simulink model "EMT_G1"  (R2024a)
settings: Solver=ode1  StartTime=0.0  StopTime=simtime  FixedStep=Ts  RelTol=1e-3
values from neighbouring files (symbols this model uses):
  c0 = c0_hawk    (= 6.37282e-09)    [EMT_Phasor_parameters.m]
  c1 = c1_hawk    (= 8.76156e-09)    [EMT_Phasor_parameters.m]
  fg = 50    [EMT_Phasor_parameters.m]
  G1gen = 0.1245    [EMT_Phasor_parameters.m]
  G2gen = 0.30    (= 0.3)    [EMT_Phasor_parameters.m]
  G3gen = 0.20    (= 0.2)    [EMT_Phasor_parameters.m]
  G4sgen = 0.2078    [EMT_Phasor_parameters.m]
  G5gen = 0.20    (= 0.2)    [EMT_Phasor_parameters.m]
  G6gen = 0.2078    [EMT_Phasor_parameters.m]
  G6sgen = 0.20    (= 0.2)    [EMT_Phasor_parameters.m]
  G7gen = 0.518    [EMT_Phasor_parameters.m]
  Ihvpk = Ihv*sqrt(2)    [EMT_Phasor_parameters.m]
  l0 = l0_hawk    (= 0.00373)    [EMT_Phasor_parameters.m]
  l1 = l1_hawk    (= 0.00133)    [EMT_Phasor_parameters.m]
  L3dem = 0.10    (= 0.1)    [EMT_Phasor_parameters.m]
  L4dem = 0.30    (= 0.3)    [EMT_Phasor_parameters.m]
  L5dem = 0.35    [EMT_Phasor_parameters.m]
  L6dem = 0.15    [EMT_Phasor_parameters.m]
  L7dem = 0.10    (= 0.1)    [EMT_Phasor_parameters.m]
  Pr = Sr*PF    (= 550050000)    [EMT_Phasor_parameters.m]
  Qr = sqrt(Sr^2 - Pr^2)    [EMT_Phasor_parameters.m]
  r0 = r0_hawk    (= 0.44587)    [EMT_Phasor_parameters.m]
  r1 = r1_hawk    (= 0.12087)    [EMT_Phasor_parameters.m]
  Rtpu = Xtpu/40    (= 0.00375)    [EMT_Phasor_parameters.m]
  S1non = 400e6    (= 400000000)    [EMT_Phasor_parameters.m]
  S2non = 300e6    (= 300000000)    [EMT_Phasor_parameters.m]
  S3non = 200e6    (= 200000000)    [EMT_Phasor_parameters.m]
  S4snon = 200e6    (= 200000000)    [EMT_Phasor_parameters.m]
  S5non = 500e6    (= 500000000)    [EMT_Phasor_parameters.m]
  S6non = 400e6    (= 400000000)    [EMT_Phasor_parameters.m]
  S6snon = 200e6    (= 200000000)    [EMT_Phasor_parameters.m]
  S7non = 200e6    (= 200000000)    [EMT_Phasor_parameters.m]
  simtime = 5    [EMT_Phasor_parameters.m]
  tonvsc = 0.01    [EMT_Phasor_parameters.m]
  Ts = 150e-6    (= 0.00015)    [EMT_Phasor_parameters.m]
  Vhv = 220e3    (= 220000)    [EMT_Phasor_parameters.m]
  Vmv = 22e3    (= 22000)    [EMT_Phasor_parameters.m]
  wc1 = wsw1/10    (= 848.230016469)    [EMT_Phasor_parameters.m]
  wdc1 = wc1/10    (= 84.8230016469)    [EMT_Phasor_parameters.m]
  wpq1 = wc1/10    (= 84.8230016469)    [EMT_Phasor_parameters.m]
  wsw1 = ksw1*2*pi*fg    (= 8482.30016469)    [EMT_Phasor_parameters.m]
  Xtpu = 0.15    [EMT_Phasor_parameters.m]
undefined symbols (not defined in the file or in its folder): D11, Delta, Kf, r, theta0
libraries: simulink_extras x152, spsGroundLib x45, powerlib x40, spsCurrentMeasurementLib x39, spsVoltageMeasurementLib x33, simulink x32, eeGeneralControl x32, slpidlib x32, powerlib_meascontrol x28, spsFirstOrderFilterLib x24, eeTransforms x24, pid_lib x16
(part 4 of 16)

== system EMT_G1/G5/VSC ==
  note: If using different transformer connection,
      | compensate the delay in the modulation
  Block : Step  Time=0.02  Before=1  After=0  SampleTime=0
  NOT : Logic  Operator=NOT  IconShape=distinctive  AllPortsSameDT=off  OutDataTypeStr=boolean
  Pset : Step  Time=tonvsc  After=-S5non*G5gen  SampleTime=0
  Qset : Step  Time=tonvsc  After=-30e6  SampleTime=0
  Three-Phase Transformer (Two Windings) : spsThreePhaseTransformerTwoWindingsLib/Three-Phase Transformer (Two Windings)  Winding1Connection=Yg  Winding2Connection=Delta (D11)  CoreType=Three single-phase transformers  SetSaturation=off  Hysteresis=off  DataFile='hysteresis'  SetInitialFlux=off  Measurements=None  UNITS=pu  NominalPower=[Pconv , fg ]  Winding1=[Vhv, Rtpu/2, Xtpu/2]  Winding2=[Vmv, Rtpu/2, Xtpu/2]  Rm=5000  Lm=5000  L0=0.5  Saturation=[ 0,0 ; 0.0024,1.2 ; 1.0,1.52 ]  InitialFluxes=[ 0.8 , -0.8 , 0.7 ]  BreakLoop=off  DiscreteSolver=Trapezoidal iterative  DataType=off  TransfoNumber=1
  Three-Phase Breaker : spsThreePhaseBreakerLib/Three-Phase Breaker  InitialState=open  SwitchA=on  SwitchB=on  SwitchC=on  SwitchTimes="[1/60  5/60]"  External=on  BreakerResistance=0.001  SnubberResistance=1e7  SnubberCapacitance=inf  Measurements=None
  VI measurement : Subsystem
      settings: PortSchema="{\"entries\":[{\"content\":{\"sides\":[{\"content\":{\"connectorIds\":[\"LConn1\",\"LConn2\",\"LConn3\"]},\"type\":\"ConnectorPlacement.EquallySpacedRectSide\",\"uuid\":\"d0d5b0b8-afec-4f90-9eba-536a06b10059\"},{\"content\":{\"connectorIds\":[\"RConn1\",\"RConn2\",\"RConn3\"],\"side\":\"RIGHT\"},\"type\":\"ConnectorPlacement.EquallySpacedRectSide\",\"uuid\":\"adc1b68d-6172-4507-b54b-9373921355a1\"},{\"content\":{\"connectorIds\":[\"Out1\",\"Out2\"],\"side\":\"TOP\"},\"type\":\"ConnectorPlacement.EquallySpacedRectSide\",\"uuid\":\"8c5adf07-e95b-4907-94c3-1b2a47d47f40\"}]},\"type\":\"ConnectorPlacement.EquallySpacedConnector\",\"uuid\":\"87d0b20f-8f85-4790-a611-3415e642a83a\"}],\"packageUris\":[\"http://schema.mathworks.com/mf0/Connector/R2020b\"],\"version\":\"1.0\"}"
  VSC Control : Subsystem
      settings: PortSchema="{\"entries\":[{\"content\":{\"sides\":[{\"content\":{\"connectorIds\":[\"In1\",\"In2\",\"In3\",\"In4\",\"In5\"]},\"type\":\"ConnectorPlacement.EquallySpacedRectSide\",\"uuid\":\"cada8d9e-53e0-4197-9386-6c7b6ea13844\"},{\"content\":{\"connectorIds\":[\"Out1\"],\"side\":\"RIGHT\"},\"type\":\"ConnectorPlacement.EquallySpacedRectSide\",\"uuid\":\"f237b52a-0d77-45c0-937d-32cafba1283e\"},{\"content\":{\"connectorIds\":[\"Out2\"],\"side\":\"TOP\"},\"type\":\"ConnectorPlacement.EquallySpacedRectSide\",\"uuid\":\"e6f268b5-5f09-49a6-9529-b1aeebd5f021\"}]},\"type\":\"ConnectorPlacement.EquallySpacedConnector\",\"uuid\":\"4d1d2957-2eb9-4111-8c87-957e800b2b0b\"}],\"packageUris\":[\"http://schema.mathworks.com/mf0/Connector/19700101\"],\"version\":\"1.0\"}"
  VSC Model : Subsystem  Variant=on  VariantControlMode=label  LabelModeActiveChoice=EMT_AVG
      settings: PortSchema="{\"entries\":[{\"content\":{\"sides\":[{\"content\":{\"connectorIds\":[\"LConn1\",\"LConn2\",\"LConn3\"]},\"type\":\"ConnectorPlacement.EquallySpacedRectSide\",\"uuid\":\"96043b84-a665-4cb2-a938-d6633d7ee474\"},{\"content\":{\"connectorIds\":[\"In1\"],\"side\":\"RIGHT\"},\"type\":\"ConnectorPlacement.EquallySpacedRectSide\",\"uuid\":\"064d463f-c23a-42ac-89ce-8dea3d446214\"},{\"content\":{\"connectorIds\":[],\"side\":\"TOP\"},\"type\":\"ConnectorPlacement.EquallySpacedRectSide\",\"uuid\":\"95ef669c-c6ed-44c3-8b69-447906728b6d\"}]},\"type\":\"ConnectorPlacement.EquallySpacedConnector\",\"uuid\":\"ea66db09-64d7-4d7e-ba7b-d769c56e2dbd\"}],\"packageUris\":[\"http://schema.mathworks.com/mf0/Connector/19700101\"],\"version\":\"1.0\"}"
  output signals : Subsystem
  A : PMIOPort  Side=Left
  B : PMIOPort  Port=2  Side=Left
  C : PMIOPort  Port=3  Side=Left
  m : Outport
  wires:
  NOT/1 -> Three-Phase Breaker/1
  VSC Control/1(Ref) -> VSC Model/1(Ref)
  [Is] -> VSC Control/3(Iabc)
  [Vs] -> VSC Control/2(Vabc)
  Block/1 -> VSC Control/1(Block), NOT/1
  [Vs] -> output signals/1(Vs)
  [Is] -> output signals/2(Is)
  VSC Control/2(m) -> output signals/3(control)
  output signals/1(m) -> m/1
  VI measurement/1(Vs) -> [Vs]
  VI measurement/2(Is) -> [Is]
  Pset/1 -> VSC Control/4(Pset)
  Qset/1 -> VSC Control/5(Qset)
  connections:
  Three-Phase Transformer (Two Windings)/LConn3 -- Three-Phase Breaker/LConn3
  Three-Phase Transformer (Two Windings)/LConn2 -- Three-Phase Breaker/LConn2
  Three-Phase Transformer (Two Windings)/LConn1 -- Three-Phase Breaker/LConn1
  Three-Phase Transformer (Two Windings)/RConn3 -- VSC Model/LConn3
  Three-Phase Transformer (Two Windings)/RConn2 -- VSC Model/LConn2
  Three-Phase Transformer (Two Windings)/RConn1 -- VSC Model/LConn1
  Three-Phase Breaker/RConn1 -- VI measurement/RConn1
  Three-Phase Breaker/RConn2 -- VI measurement/RConn2
  Three-Phase Breaker/RConn3 -- VI measurement/RConn3
  VI measurement/LConn3 -- C/RConn1
  A/RConn1 -- VI measurement/LConn1
  B/RConn1 -- VI measurement/LConn2

== system EMT_G1/G6/VSC ==
  note: If using different transformer connection,
      | compensate the delay in the modulation
  Block : Step  Time=0.02  Before=1  After=0  SampleTime=0
  NOT : Logic  Operator=NOT  IconShape=distinctive  AllPortsSameDT=off  OutDataTypeStr=boolean
  Pset : Step  Time=tonvsc  After=-S6non*G6gen  SampleTime=0
  Qset : Step  Time=tonvsc  After=-30e6  SampleTime=0
  Three-Phase Transformer (Two Windings) : spsThreePhaseTransformerTwoWindingsLib/Three-Phase Transformer (Two Windings)  Winding1Connection=Yg  Winding2Connection=Delta (D11)  CoreType=Three single-phase transformers  SetSaturation=off  Hysteresis=off  DataFile='hysteresis'  SetInitialFlux=off  Measurements=None  UNITS=pu  NominalPower=[Pconv , fg ]  Winding1=[Vhv, Rtpu/2, Xtpu/2]  Winding2=[Vmv, Rtpu/2, Xtpu/2]  Rm=5000  Lm=5000  L0=0.5  Saturation=[ 0,0 ; 0.0024,1.2 ; 1.0,1.52 ]  InitialFluxes=[ 0.8 , -0.8 , 0.7 ]  BreakLoop=off  DiscreteSolver=Trapezoidal iterative  DataType=off  TransfoNumber=1
  Three-Phase Breaker : spsThreePhaseBreakerLib/Three-Phase Breaker  InitialState=open  SwitchA=on  SwitchB=on  SwitchC=on  SwitchTimes="[1/60  5/60]"  External=on  BreakerResistance=0.001  SnubberResistance=1e7  SnubberCapacitance=inf  Measurements=None
  VI measurement : Subsystem
      settings: PortSchema="{\"entries\":[{\"content\":{\"sides\":[{\"content\":{\"connectorIds\":[\"LConn1\",\"LConn2\",\"LConn3\"]},\"type\":\"ConnectorPlacement.EquallySpacedRectSide\",\"uuid\":\"d0d5b0b8-afec-4f90-9eba-536a06b10059\"},{\"content\":{\"connectorIds\":[\"RConn1\",\"RConn2\",\"RConn3\"],\"side\":\"RIGHT\"},\"type\":\"ConnectorPlacement.EquallySpacedRectSide\",\"uuid\":\"adc1b68d-6172-4507-b54b-9373921355a1\"},{\"content\":{\"connectorIds\":[\"Out1\",\"Out2\"],\"side\":\"TOP\"},\"type\":\"ConnectorPlacement.EquallySpacedRectSide\",\"uuid\":\"8c5adf07-e95b-4907-94c3-1b2a47d47f40\"}]},\"type\":\"ConnectorPlacement.EquallySpacedConnector\",\"uuid\":\"87d0b20f-8f85-4790-a611-3415e642a83a\"}],\"packageUris\":[\"http://schema.mathworks.com/mf0/Connector/R2020b\"],\"version\":\"1.0\"}"
  VSC Control : Subsystem
      settings: PortSchema="{\"entries\":[{\"content\":{\"sides\":[{\"content\":{\"connectorIds\":[\"In1\",\"In2\",\"In3\",\"In4\",\"In5\"]},\"type\":\"ConnectorPlacement.EquallySpacedRectSide\",\"uuid\":\"cada8d9e-53e0-4197-9386-6c7b6ea13844\"},{\"content\":{\"connectorIds\":[\"Out1\"],\"side\":\"RIGHT\"},\"type\":\"ConnectorPlacement.EquallySpacedRectSide\",\"uuid\":\"f237b52a-0d77-45c0-937d-32cafba1283e\"},{\"content\":{\"connectorIds\":[\"Out2\"],\"side\":\"TOP\"},\"type\":\"ConnectorPlacement.EquallySpacedRectSide\",\"uuid\":\"e6f268b5-5f09-49a6-9529-b1aeebd5f021\"}]},\"type\":\"ConnectorPlacement.EquallySpacedConnector\",\"uuid\":\"4d1d2957-2eb9-4111-8c87-957e800b2b0b\"}],\"packageUris\":[\"http://schema.mathworks.com/mf0/Connector/19700101\"],\"version\":\"1.0\"}"
  VSC Model : Subsystem  Variant=on  VariantControlMode=label  LabelModeActiveChoice=EMT_AVG
      settings: PortSchema="{\"entries\":[{\"content\":{\"sides\":[{\"content\":{\"connectorIds\":[\"LConn1\",\"LConn2\",\"LConn3\"]},\"type\":\"ConnectorPlacement.EquallySpacedRectSide\",\"uuid\":\"96043b84-a665-4cb2-a938-d6633d7ee474\"},{\"content\":{\"connectorIds\":[\"In1\"],\"side\":\"RIGHT\"},\"type\":\"ConnectorPlacement.EquallySpacedRectSide\",\"uuid\":\"064d463f-c23a-42ac-89ce-8dea3d446214\"},{\"content\":{\"connectorIds\":[],\"side\":\"TOP\"},\"type\":\"ConnectorPlacement.EquallySpacedRectSide\",\"uuid\":\"95ef669c-c6ed-44c3-8b69-447906728b6d\"}]},\"type\":\"ConnectorPlacement.EquallySpacedConnector\",\"uuid\":\"ea66db09-64d7-4d7e-ba7b-d769c56e2dbd\"}],\"packageUris\":[\"http://schema.mathworks.com/mf0/Connector/19700101\"],\"version\":\"1.0\"}"
  output signals : Subsystem
  A : PMIOPort  Side=Left
  B : PMIOPort  Port=2  Side=Left
  C : PMIOPort  Port=3  Side=Left
  m : Outport
  wires:
  NOT/1 -> Three-Phase Breaker/1
  VSC Control/1(Ref) -> VSC Model/1(Ref)
  [Is] -> VSC Control/3(Iabc)
  [Vs] -> VSC Control/2(Vabc)
  Block/1 -> VSC Control/1(Block), NOT/1
  [Vs] -> output signals/1(Vs)
  [Is] -> output signals/2(Is)
  VSC Control/2(m) -> output signals/3(control)
  output signals/1(m) -> m/1
  VI measurement/1(Vs) -> [Vs]
  VI measurement/2(Is) -> [Is]
  Pset/1 -> VSC Control/4(Pset)
  Qset/1 -> VSC Control/5(Qset)
  connections:
  Three-Phase Transformer (Two Windings)/LConn3 -- Three-Phase Breaker/LConn3
  Three-Phase Transformer (Two Windings)/LConn2 -- Three-Phase Breaker/LConn2
  Three-Phase Transformer (Two Windings)/LConn1 -- Three-Phase Breaker/LConn1
  Three-Phase Transformer (Two Windings)/RConn3 -- VSC Model/LConn3
  Three-Phase Transformer (Two Windings)/RConn2 -- VSC Model/LConn2
  Three-Phase Transformer (Two Windings)/RConn1 -- VSC Model/LConn1
  Three-Phase Breaker/RConn1 -- VI measurement/RConn1
  Three-Phase Breaker/RConn2 -- VI measurement/RConn2
  Three-Phase Breaker/RConn3 -- VI measurement/RConn3
  VI measurement/LConn3 -- C/RConn1
  A/RConn1 -- VI measurement/LConn1
  B/RConn1 -- VI measurement/LConn2

== system EMT_G1/G6s/Exciter System ==
  <dw> : Inport
  Vref : Inport  Port=2
  Vt : Inport  Port=3
  It : Inport  Port=4
  <Peo> : Inport  Port=5
  PSS : Subsystem  mask{Ks1=10, Ks2=0.1564, Ks3=1, Tw1=2, Tw2=2, Tw3=2, Tw4=0, T1=0.25, T2=0.03, T3=0.15, T4=0.015, T6=0, T7=2, T8=0.5, T9=0.1, Vstmin=-0.1, Vstmax=0.1, N=0, M=0, IC1=1, IC2=3}
      mask prompts: Ks1 "PSS gain (Ks1)"; Ks2 "2nd signal transducer factor(Ks2)"; Ks3 "washouts coupling factor (Ks3)"; Tw1 "1st washout 1th time constant (Tw1)(sec)"; Tw2 "1st washout 2nd time constant (Tw2)(sec)"; Tw3 "2nd washout 1st time constant (Tw3)(sec)"; Tw4 "2nd washout 2nd time constant (Tw4)(sec)"; T1 "1st lead-lag derivative time constant (T1)(sec)"; T2 "1st lead-lag delay time constant(T2)(sec)"; T3 "2nd lead-lag derivative time constant(T3)(sec)"; T4 "2nd lead-lag delay time constant(T4)(sec)"; T6 "1st signal transducer time constant(T6)(sec)"; T7 "2nd signal transducer time constant(T7)(sec)"; T8 "ramp tracking filter deriv. time constant(T8)(sec)"; T9 "ramp tracking filter delay time constant(T9)(sec)"; Vstmin "controller minimum output(Vstmin)"; Vstmax "controller maximum output(Vstmax)"; N "ramp tracking filter (N)"; M "ramp tracking filter (M)"; IC1 "1st input selector (IC1)"; IC2 "2nd input selector (IC2)"
      mask Display:
      | disp('PSS2A')
      | 
      | port_label('input',1,'dw')
      | port_label('input',2,'Pg')
      | %port_label('input',3,'Vs')
      | 
      | port_label('output',1,'Vs')
  SEXS : Subsystem  mask{K=200, Ta=3, Tb=10, Te=0.05, Emin=-4, Emax=4, Vf0=1.68751}
      mask prompts: K "Controller gain (K)"; Ta "Filter derivative time constant (Ta)(sec)"; Tb "Filter delay time (Tb)(sec)"; Te "Exciter time constant (Te)(sec)"; Emin "Controller minimum output (Emin)"; Emax "Controller maximum output (Emax)"; Vf0 "Initial output (p.u)"
      mask Display:
      | disp('AVR')
      | 
      | port_label('input',1,'Vref')
      | port_label('input',2,'Vc')
      | port_label('input',3,'Vs')
      | 
      | port_label('output',1,'Efd')
  TR and LC_test : Subsystem  mask{Tr=1e-3, Rc=0, Xc=0}
      mask prompts: Tr "Transducter filter time constant (Tr)(sec)"; Rc "Resistance to compensate (p.u)"; Xc "Reactance to compensate (p.u)"
      mask Display:
      | %disp('Transducer \n \n')
      | %disp('and \n')
      | %disp('Load compensation')
      | text(15,35, 'Transducer')
      | text(30,24, 'and')
      | text(15,14, 'Load comp')
      | 
      | port_label('input',1,'Vt')
      | port_label('input',2,'It')
      | 
      | port_label('output',1,'Vc')
  Efd : Outport
  wires:
  SEXS/1(Efd) -> Efd/1
  It/1 -> TR and LC_test/2(It)
  PSS/1(Vothsg) -> SEXS/3(Vs)
  <Peo>/1 -> PSS/2(Pgen)
  <dw>/1 -> PSS/1(dw)
  Vt/1 -> TR and LC_test/1(Vt)
  Vref/1 -> SEXS/1(Vref)
  TR and LC_test/1(Vc) -> SEXS/2(Vc)

== system EMT_G1/G6s/Speed Governor ==
  note: mechanical power
  RefL : Inport
  dw : Inport  Port=2
  Gain1 : Gain  Gain=Dt
  Gain2 : Gain  Gain=1/R
  Saturation : Saturate  UpperLimit=Vmax  LowerLimit=Vmin
  Saturation1 : Saturate  UpperLimit=1
  Scope : Scope  NumInputPorts=2
  Sum : Sum  Inputs=|+-
  Sum1 : Sum  Inputs=|+-
  Transfer Fcn (with initial outputs)1 : simulink_extras/Additional Linear/Transfer Fcn (with initial outputs)  N=[T2 1]  D=[T3 1]  Y0=P0  U0=P0
  Transfer Fcn (with initial outputs)2 : simulink_extras/Additional Linear/Transfer Fcn (with initial outputs)  N=[1]  D=[T1 1]  Y0=P0  U0=P0
  Pm : Outport
  wires:
  Gain2/1 -> Sum/2
  dw/1 -> Gain2/1, Gain1/1
  Gain1/1 -> Sum1/2
  Transfer Fcn (with initial outputs)1/1 -> Sum1/1
  Sum1/1 -> Saturation1/1
  Saturation/1 -> Scope/1, Transfer Fcn (with initial outputs)1/1
  Transfer Fcn (with initial outputs)2/1 -> Saturation/1
  Sum/1 -> Transfer Fcn (with initial outputs)2/1
  RefL/1 -> Sum/1
  Saturation1/1 -> Scope/2, Pm/1

== system EMT_G1/G7/Exciter System ==
  <dw> : Inport
  Vref : Inport  Port=2
  Vt : Inport  Port=3
  It : Inport  Port=4
  <Peo> : Inport  Port=5
  PSS1 : Subsystem  mask{Ks1=10, Ks2=0.1564, Ks3=1, Tw1=2, Tw2=2, Tw3=2, Tw4=0, T1=0.25, T2=0.03, T3=0.15, T4=0.015, T6=0, T7=2, T8=0.5, T9=0.1, Vstmin=-0.1, Vstmax=0.1, N=0, M=0, IC1=1, IC2=3}
      mask prompts: Ks1 "PSS gain (Ks1)"; Ks2 "2nd signal transducer factor(Ks2)"; Ks3 "washouts coupling factor (Ks3)"; Tw1 "1st washout 1th time constant (Tw1)(sec)"; Tw2 "1st washout 2nd time constant (Tw2)(sec)"; Tw3 "2nd washout 1st time constant (Tw3)(sec)"; Tw4 "2nd washout 2nd time constant (Tw4)(sec)"; T1 "1st lead-lag derivative time constant (T1)(sec)"; T2 "1st lead-lag delay time constant(T2)(sec)"; T3 "2nd lead-lag derivative time constant(T3)(sec)"; T4 "2nd lead-lag delay time constant(T4)(sec)"; T6 "1st signal transducer time constant(T6)(sec)"; T7 "2nd signal transducer time constant(T7)(sec)"; T8 "ramp tracking filter deriv. time constant(T8)(sec)"; T9 "ramp tracking filter delay time constant(T9)(sec)"; Vstmin "controller minimum output(Vstmin)"; Vstmax "controller maximum output(Vstmax)"; N "ramp tracking filter (N)"; M "ramp tracking filter (M)"; IC1 "1st input selector (IC1)"; IC2 "2nd input selector (IC2)"
      mask Display:
      | disp('PSS2A')
      | 
      | port_label('input',1,'dw')
      | port_label('input',2,'Pg')
      | %port_label('input',3,'Vs')
      | 
      | port_label('output',1,'Vs')
  SEXS : Subsystem  mask{K=200, Ta=3, Tb=10, Te=0.05, Emin=-4, Emax=4, Vf0=1.77627}
      mask prompts: K "Controller gain (K)"; Ta "Filter derivative time constant (Ta)(sec)"; Tb "Filter delay time (Tb)(sec)"; Te "Exciter time constant (Te)(sec)"; Emin "Controller minimum output (Emin)"; Emax "Controller maximum output (Emax)"; Vf0 "Initial output (p.u)"
      mask Display:
      | disp('AVR')
      | 
      | port_label('input',1,'Vref')
      | port_label('input',2,'Vc')
      | port_label('input',3,'Vs')
      | 
      | port_label('output',1,'Efd')
  TR and LC_test : Subsystem  mask{Tr=1e-3, Rc=0, Xc=0}
      mask prompts: Tr "Transducter filter time constant (Tr)(sec)"; Rc "Resistance to compensate (p.u)"; Xc "Reactance to compensate (p.u)"
      mask Display:
      | %disp('Transducer \n \n')
      | %disp('and \n')
      | %disp('Load compensation')
      | text(15,35, 'Transducer')
      | text(30,24, 'and')
      | text(15,14, 'Load comp')
      | 
      | port_label('input',1,'Vt')
      | port_label('input',2,'It')
      | 
      | port_label('output',1,'Vc')
  Efd : Outport
  wires:
  TR and LC_test/1(Vc) -> SEXS/2(Vc)
  Vref/1 -> SEXS/1(Vref)
  Vt/1 -> TR and LC_test/1(Vt)
  <dw>/1 -> PSS1/1(dw)
  <Peo>/1 -> PSS1/2(Pgen)
  PSS1/1(Vothsg) -> SEXS/3(Vs)
  It/1 -> TR and LC_test/2(It)
  SEXS/1(Efd) -> Efd/1

== system EMT_G1/G7/Speed Governor ==
  note: mechanical power
  RefL : Inport
  dw : Inport  Port=2
  Gain1 : Gain  Gain=Dt
  Gain2 : Gain  Gain=1/R
  Saturation : Saturate  UpperLimit=Vmax  LowerLimit=Vmin
  Saturation1 : Saturate  UpperLimit=1
  Sum : Sum  Inputs=|+-
  Sum1 : Sum  Inputs=|+-
  Transfer Fcn (with initial outputs)1 : simulink_extras/Additional Linear/Transfer Fcn (with initial outputs)  N=[T2 1]  D=[T3 1]  Y0=P0  U0=P0
  Transfer Fcn (with initial outputs)2 : simulink_extras/Additional Linear/Transfer Fcn (with initial outputs)  N=[1]  D=[T1 1]  Y0=P0  U0=P0
  Pm : Outport
  wires:
  Saturation1/1 -> Pm/1
  RefL/1 -> Sum/1
  Sum/1 -> Transfer Fcn (with initial outputs)2/1
  Transfer Fcn (with initial outputs)2/1 -> Saturation/1
  Saturation/1 -> Transfer Fcn (with initial outputs)1/1
  Sum1/1 -> Saturation1/1
  Transfer Fcn (with initial outputs)1/1 -> Sum1/1
  Gain1/1 -> Sum1/2
  dw/1 -> Gain1/1, Gain2/1
  Gain2/1 -> Sum/2

== system EMT_G1/G1/Exciter System/PSS1 ==
  note: Power System Stabilizer (PSS2A)
  dw : Inport
  Pgen : Inport  Port=2
  Gain : Gain  Gain=Ks1
  Gain1 : Gain  Gain=Ks3
  Saturation : Saturate  UpperLimit=Vstmax  LowerLimit=Vstmin
  Sum1 : Sum  Inputs=|++
  Sum2 : Sum  Inputs=|+-
  Transfer Fcn1 : TransferFcn  Numerator=[Tw1 0]  Denominator=[Tw1 1]
  Transfer Fcn2 : TransferFcn  Numerator=[Tw3 0]  Denominator=[Tw3 1]
  Transfer Fcn3 : TransferFcn  Numerator=[Tw2 0]  Denominator=[Tw2 1]
  Transfer Fcn4 : TransferFcn  Denominator=[T6 1]
  Transfer Fcn5 : TransferFcn  Numerator=[T8 1].^N  Denominator=[T9 1].^(M*N)
  Transfer Fcn6 : TransferFcn  Numerator=[T1 1]  Denominator=[T2 1]
  Transfer Fcn7 : TransferFcn  Numerator=[T3 1]  Denominator=[T4 1]
  Transfer Fcn8 : TransferFcn  Numerator=[Tw4 0]  Denominator=[Tw4 1]
  Transfer Fcn9 : TransferFcn  Numerator=[Ks2]  Denominator=[T7 1]
  Vothsg : Outport
  wires:
  dw/1 -> Transfer Fcn1/1
  Transfer Fcn1/1 -> Transfer Fcn3/1
  Transfer Fcn3/1 -> Transfer Fcn4/1
  Transfer Fcn4/1 -> Sum1/1
  Sum1/1 -> Transfer Fcn5/1
  Transfer Fcn5/1 -> Sum2/1
  Sum2/1 -> Gain/1
  Gain/1 -> Transfer Fcn6/1
  Transfer Fcn6/1 -> Transfer Fcn7/1
  Transfer Fcn7/1 -> Saturation/1
  Saturation/1 -> Vothsg/1
  Pgen/1 -> Transfer Fcn2/1
  Transfer Fcn2/1 -> Transfer Fcn8/1
  Transfer Fcn8/1 -> Transfer Fcn9/1
  Gain1/1 -> Sum1/2
  Transfer Fcn9/1 -> Gain1/1, Sum2/2

== system EMT_G1/G1/Exciter System/PSS1 backup ==
  note: Power System Stabilizer (PSS2A)
  dw : Inport
  Pgen : Inport  Port=2
  Gain : Gain  Gain=Ks1
  Gain1 : Gain  Gain=Ks3
  Saturation : Saturate  UpperLimit=Vstmax  LowerLimit=Vstmin
  Sum1 : Sum  Inputs=|++
  Sum2 : Sum  Inputs=|+-
  Transfer Fcn1 : TransferFcn  Numerator=[Tw1 0]  Denominator=[Tw1 1]
  Transfer Fcn2 : TransferFcn  Numerator=[Tw3 0]  Denominator=[Tw3 1]
  Transfer Fcn3 : TransferFcn  Numerator=[Tw2 0]  Denominator=[Tw2 1]
  Transfer Fcn4 : TransferFcn  Denominator=[T6 1]
  Transfer Fcn5 : TransferFcn  Numerator=[T8 1].^N  Denominator=[T9 1].^(M*N)
  Transfer Fcn6 : TransferFcn  Numerator=[T1 1]  Denominator=[T2 1]
  Transfer Fcn7 : TransferFcn  Numerator=[T3 1]  Denominator=[T4 1]
  Transfer Fcn8 : TransferFcn  Numerator=[Tw4 0]  Denominator=[Tw4 1]
  Transfer Fcn9 : TransferFcn  Numerator=[Ks2]  Denominator=[T7 1]
  Vothsg : Outport
  wires:
  Transfer Fcn9/1 -> Sum2/2, Gain1/1
  Gain1/1 -> Sum1/2
  Transfer Fcn8/1 -> Transfer Fcn9/1
  Transfer Fcn2/1 -> Transfer Fcn8/1
  Pgen/1 -> Transfer Fcn2/1
  Saturation/1 -> Vothsg/1
  Transfer Fcn7/1 -> Saturation/1
  Transfer Fcn6/1 -> Transfer Fcn7/1
  Gain/1 -> Transfer Fcn6/1
  Sum2/1 -> Gain/1
  Transfer Fcn5/1 -> Sum2/1
  Sum1/1 -> Transfer Fcn5/1
  Transfer Fcn4/1 -> Sum1/1
  Transfer Fcn3/1 -> Transfer Fcn4/1
  Transfer Fcn1/1 -> Transfer Fcn3/1
  dw/1 -> Transfer Fcn1/1

== system EMT_G1/G1/Exciter System/SEXS ==
  note: The controller parameters provided by ENTSO-E
      | define different names for the parameters:
      |
      | ENTSO-E = IEEE Std 421.5-2005
      | Ta = Tc
      | Tb = Tb
      | K = Ka
      | Te = Ta
      | Emax = Vrmax
      | Emin = Vrmin
  note: The exciter model provided by ENTSO-E most similar to the IEEE is the Type AC4A excitation system model
  Vref : Inport
  Vc : Inport  Port=2
  Vs : Inport  Port=3
  1st ord transfer fcn windup limiter : Subsystem  mask{Gain=K, tau=Te, Vmax=Emax, Vmin=Emin, y0=Vf0}
      mask prompts: tau "Time constant"; y0 "Initial output"
  Constant : Constant  Value=Vf0/K
  Saturation : Saturate  Commented=through  UpperLimit=0.1  LowerLimit=-0.1
  Sum : Sum  Inputs=+-+
  Sum1 : Sum  Inputs=|++
  Transfer Fcn (with initial outputs)1 : simulink_extras/Additional Linear/Transfer Fcn (with initial outputs)  N=[Ta 1]  D=[Tb 1]  Y0=Vf0/K  U0=Vf0/K
  Efd : Outport
  wires:
  1st ord transfer fcn windup limiter/1(Out1) -> Efd/1
  Vs/1 -> Sum/3
  Vref/1 -> Sum/1
  Vc/1 -> Sum/2
  Transfer Fcn (with initial outputs)1/1 -> 1st ord transfer fcn windup limiter/1(In1)
  Saturation/1 -> Transfer Fcn (with initial outputs)1/1
  Sum/1 -> Sum1/1
  Sum1/1 -> Saturation/1
  Constant/1 -> Sum1/2

== system EMT_G1/G1/Exciter System/TR and LC_test ==
  note: Terminal voltage transducer and optional load compensation
  note: compensated
      | impedance
  note: Vt and It should be phasors (complex quantities)
  note: Fig 4.1 of IEEE Std 421.5-2005
  note: Rc and Xc should be negative values in case of voltage regulated after an impedance
  Vt : Inport
  It : Inport  Port=2
  Abs : Abs  SaturateOnIntegerOverflow=off
  Abs1 : Abs  SaturateOnIntegerOverflow=off
  Rc+jXc : Gain  Gain=abs(Rc+1i*Xc)
  Saturation : Saturate  UpperLimit=1.2  LowerLimit=0.8
  Sum : Sum  Inputs=|+-
  Transfer Fcn (with initial outputs) : simulink_extras/Additional Linear/Transfer Fcn (with initial outputs)  Commented=through  N=[1]  D=[Tr 1]  Y0=1  U0=1
  Vc : Outport
  wires:
  Saturation/1 -> Vc/1
  Vt/1 -> Abs/1
  Transfer Fcn (with initial outputs)/1 -> Saturation/1
  Rc+jXc/1 -> Sum/2
  Sum/1 -> Transfer Fcn (with initial outputs)/1
  It/1 -> Abs1/1
  Abs/1 -> Sum/1
  Abs1/1 -> Rc+jXc/1

== system EMT_G1/G2/VSC/VI measurement ==
  Current Measurement : spsCurrentMeasurementLib/Current Measurement  PhasorSimulation=off  OutputType=Complex  PSBequivalent=0
  Current Measurement1 : spsCurrentMeasurementLib/Current Measurement  PhasorSimulation=off  OutputType=Complex  PSBequivalent=0
  Current Measurement2 : spsCurrentMeasurementLib/Current Measurement  PhasorSimulation=off  OutputType=Complex  PSBequivalent=0
  Ground : spsGroundLib/Ground  LConnTagsString=a
  Ground1 : spsGroundLib/Ground  LConnTagsString=a
  Ground2 : spsGroundLib/Ground  LConnTagsString=a
  Mux : Mux  Inputs=3
  Mux1 : Mux  Inputs=3
  Voltage Measurement : spsVoltageMeasurementLib/Voltage Measurement  PhasorSimulation=off  OutputType=Complex  PSBequivalent=0
  Voltage Measurement1 : spsVoltageMeasurementLib/Voltage Measurement  PhasorSimulation=off  OutputType=Complex  PSBequivalent=0
  Voltage Measurement2 : spsVoltageMeasurementLib/Voltage Measurement  PhasorSimulation=off  OutputType=Complex  PSBequivalent=0
  A : PMIOPort  Side=Left
  B : PMIOPort  Port=2  Side=Left
  C : PMIOPort  Port=3  Side=Left
  a : PMIOPort  Port=4  Side=Right
  b : PMIOPort  Port=5  Side=Right
  c : PMIOPort  Port=6  Side=Right
  Vs : Outport
  Is : Outport  Port=2
  wires:
  Mux1/1 -> Is/1
  Mux/1 -> Vs/1
  Voltage Measurement1/1 -> Mux/2
  Voltage Measurement2/1 -> Mux/3
  Current Measurement2/1 -> Mux1/3
  Voltage Measurement/1 -> Mux/1
  Current Measurement/1 -> Mux1/1
  Current Measurement1/1 -> Mux1/2
  connections:
  Voltage Measurement/LConn1 -- Current Measurement/LConn1 -- A/RConn1
  Current Measurement2/LConn1 -- C/RConn1 -- Voltage Measurement2/LConn1
  Current Measurement1/LConn1 -- Voltage Measurement1/LConn1 -- B/RConn1
  Current Measurement1/RConn1 -- b/RConn1
  Current Measurement/RConn1 -- a/RConn1
  Ground/LConn1 -- Voltage Measurement/LConn2
  Current Measurement2/RConn1 -- c/RConn1
  Ground1/LConn1 -- Voltage Measurement1/LConn2
  Ground2/LConn1 -- Voltage Measurement2/LConn2

== system EMT_G1/G2/VSC/VSC Control ==
  Block : Inport
  Vabc : Inport  Port=2
  Iabc : Inport  Port=3
  Pset : Inport  Port=4
  Qset : Inport  Port=5
  Control loops : Subsystem  Variant=on  VariantControlMode=label  LabelModeActiveChoice=EMT_and_QEMT
  Measurements : Subsystem  Variant=on  VariantControlMode=label  LabelModeActiveChoice=EMT
  Modulation : Subsystem  Variant=on  VariantControlMode=label  LabelModeActiveChoice=EMT_AVG
  Mux : Mux  Inputs=2
  Ref : Outport
  m : Outport  Port=2
  wires:
  Control loops/2(iqd+-ref) -> Modulation/3(iqd+-*)
  Control loops/1(vqd+-ref) -> Modulation/2(vqd+-*)
  [PQabc] -> Mux/2
  Measurements/5(PQabc) -> [PQabc]
  Modulation/1(Ref) -> Ref/1
  Measurements/4(theta) -> [theta]
  Vabc/1 -> Measurements/1(Vabc)
  Measurements/1(vqd+-) -> Control loops/3(vqd+-), [vqdpn]
  Measurements/2(iqd+-) -> Control loops/4(iqd+-)
  Measurements/3(freq) -> Control loops/5(freq)
  [theta] -> Modulation/4(theta)
  [vqdpn] -> Modulation/1(vqd+-)
  Iabc/1 -> Measurements/2(Iabc)
  Mux/1 -> m/1
  Control loops/3(m) -> Mux/1
  Pset/1 -> Control loops/1(Pset)
  Qset/1 -> Control loops/2(Qset)
  Block/1 -> Control loops/6(Block)

== system EMT_G1/G2/VSC/VSC Model ==
  Ref : Inport
  EMT AVG : Subsystem  VariantControl=EMT_AVG
      settings: PortSchema="{\"entries\":[{\"content\":{\"sides\":[{\"content\":{\"connectorIds\":[\"LConn1\",\"LConn2\",\"LConn3\"]},\"type\":\"ConnectorPlacement.EquallySpacedRectSide\",\"uuid\":\"96043b84-a665-4cb2-a938-d6633d7ee474\"},{\"content\":{\"connectorIds\":[\"In1\"],\"side\":\"RIGHT\"},\"type\":\"ConnectorPlacement.EquallySpacedRectSide\",\"uuid\":\"064d463f-c23a-42ac-89ce-8dea3d446214\"},{\"content\":{\"connectorIds\":[],\"side\":\"TOP\"},\"type\":\"ConnectorPlacement.EquallySpacedRectSide\",\"uuid\":\"95ef669c-c6ed-44c3-8b69-447906728b6d\"}]},\"type\":\"ConnectorPlacement.EquallySpacedConnector\",\"uuid\":\"ea66db09-64d7-4d7e-ba7b-d769c56e2dbd\"}],\"packageUris\":[\"http://schema.mathworks.com/mf0/Connector/19700101\"],\"version\":\"1.0\"}"
  EMT SW : Subsystem  VariantControl=EMT_SW
      settings: PortSchema="{\"entries\":[{\"content\":{\"sides\":[{\"content\":{\"connectorIds\":[\"LConn1\",\"LConn2\",\"LConn3\"]},\"type\":\"ConnectorPlacement.EquallySpacedRectSide\",\"uuid\":\"96043b84-a665-4cb2-a938-d6633d7ee474\"},{\"content\":{\"connectorIds\":[\"In1\"],\"side\":\"RIGHT\"},\"type\":\"ConnectorPlacement.EquallySpacedRectSide\",\"uuid\":\"064d463f-c23a-42ac-89ce-8dea3d446214\"},{\"content\":{\"connectorIds\":[],\"side\":\"TOP\"},\"type\":\"ConnectorPlacement.EquallySpacedRectSide\",\"uuid\":\"95ef669c-c6ed-44c3-8b69-447906728b6d\"}]},\"type\":\"ConnectorPlacement.EquallySpacedConnector\",\"uuid\":\"ea66db09-64d7-4d7e-ba7b-d769c56e2dbd\"}],\"packageUris\":[\"http://schema.mathworks.com/mf0/Connector/19700101\"],\"version\":\"1.0\"}"
  Phasor : Subsystem  VariantControl=Phasor
      settings: PortSchema="{\"entries\":[{\"content\":{\"sides\":[{\"content\":{\"connectorIds\":[\"LConn1\",\"LConn2\",\"LConn3\"]},\"type\":\"ConnectorPlacement.EquallySpacedRectSide\",\"uuid\":\"96043b84-a665-4cb2-a938-d6633d7ee474\"},{\"content\":{\"connectorIds\":[\"In1\"],\"side\":\"RIGHT\"},\"type\":\"ConnectorPlacement.EquallySpacedRectSide\",\"uuid\":\"064d463f-c23a-42ac-89ce-8dea3d446214\"},{\"content\":{\"connectorIds\":[],\"side\":\"TOP\"},\"type\":\"ConnectorPlacement.EquallySpacedRectSide\",\"uuid\":\"95ef669c-c6ed-44c3-8b69-447906728b6d\"}]},\"type\":\"ConnectorPlacement.EquallySpacedConnector\",\"uuid\":\"ea66db09-64d7-4d7e-ba7b-d769c56e2dbd\"}],\"packageUris\":[\"http://schema.mathworks.com/mf0/Connector/19700101\"],\"version\":\"1.0\"}"
  A : PMIOPort  Side=Left
  B : PMIOPort  Port=2  Side=Left
  C : PMIOPort  Port=3  Side=Left

== system EMT_G1/G2/VSC/output signals ==
  Vs : Inport
  Is : Inport  Port=2
  control : Inport  Port=3
  Bus Creator : BusCreator  Inputs=15
  Demux : Demux  Outputs=13
  m : Outport
  wires:
  Bus Creator/1 -> m/1
  control/1 -> Demux/1
  Vs/1 -> Bus Creator/1  "Vabc"
  Is/1 -> Bus Creator/2  "Iabc"
  Demux/1 -> Bus Creator/3  "vqp"
  Demux/2 -> Bus Creator/4  "vdp"
  Demux/3 -> Bus Creator/5  "vqn"
  Demux/4 -> Bus Creator/6  "vdn"
  Demux/5 -> Bus Creator/7  "iqp"
  Demux/6 -> Bus Creator/8  "idp"
  Demux/7 -> Bus Creator/9  "iqn"
  Demux/8 -> Bus Creator/10  "idn"
  Demux/9 -> Bus Creator/11  "f"
  Demux/10 -> Bus Creator/12  "Pdq"
  Demux/11 -> Bus Creator/13  "Qdq"
  Demux/12 -> Bus Creator/14  "Pabc"
  Demux/13 -> Bus Creator/15  "Qabc"

== system EMT_G1/G3/VSC/VI measurement ==
  Current Measurement : spsCurrentMeasurementLib/Current Measurement  PhasorSimulation=off  OutputType=Complex  PSBequivalent=0
  Current Measurement1 : spsCurrentMeasurementLib/Current Measurement  PhasorSimulation=off  OutputType=Complex  PSBequivalent=0
  Current Measurement2 : spsCurrentMeasurementLib/Current Measurement  PhasorSimulation=off  OutputType=Complex  PSBequivalent=0
  Ground : spsGroundLib/Ground  LConnTagsString=a
  Ground1 : spsGroundLib/Ground  LConnTagsString=a
  Ground2 : spsGroundLib/Ground  LConnTagsString=a
  Mux : Mux  Inputs=3
  Mux1 : Mux  Inputs=3
  Voltage Measurement : spsVoltageMeasurementLib/Voltage Measurement  PhasorSimulation=off  OutputType=Complex  PSBequivalent=0
  Voltage Measurement1 : spsVoltageMeasurementLib/Voltage Measurement  PhasorSimulation=off  OutputType=Complex  PSBequivalent=0
  Voltage Measurement2 : spsVoltageMeasurementLib/Voltage Measurement  PhasorSimulation=off  OutputType=Complex  PSBequivalent=0
  A : PMIOPort  Side=Left
  B : PMIOPort  Port=2  Side=Left
  C : PMIOPort  Port=3  Side=Left
  a : PMIOPort  Port=4  Side=Right
  b : PMIOPort  Port=5  Side=Right
  c : PMIOPort  Port=6  Side=Right
  Vs : Outport
  Is : Outport  Port=2
  wires:
  Mux1/1 -> Is/1
  Mux/1 -> Vs/1
  Voltage Measurement1/1 -> Mux/2
  Voltage Measurement2/1 -> Mux/3
  Current Measurement2/1 -> Mux1/3
  Voltage Measurement/1 -> Mux/1
  Current Measurement/1 -> Mux1/1
  Current Measurement1/1 -> Mux1/2
  connections:
  Voltage Measurement/LConn1 -- Current Measurement/LConn1 -- A/RConn1
  Current Measurement2/LConn1 -- C/RConn1 -- Voltage Measurement2/LConn1
  Current Measurement1/LConn1 -- Voltage Measurement1/LConn1 -- B/RConn1
  Current Measurement1/RConn1 -- b/RConn1
  Current Measurement/RConn1 -- a/RConn1
  Ground/LConn1 -- Voltage Measurement/LConn2
  Current Measurement2/RConn1 -- c/RConn1
  Ground1/LConn1 -- Voltage Measurement1/LConn2
  Ground2/LConn1 -- Voltage Measurement2/LConn2

== system EMT_G1/G3/VSC/VSC Control ==
  Block : Inport
  Vabc : Inport  Port=2
  Iabc : Inport  Port=3
  Pset : Inport  Port=4
  Qset : Inport  Port=5
  Control loops : Subsystem  Variant=on  VariantControlMode=label  LabelModeActiveChoice=EMT_and_QEMT
  Measurements : Subsystem  Variant=on  VariantControlMode=label  LabelModeActiveChoice=EMT
  Modulation : Subsystem  Variant=on  VariantControlMode=label  LabelModeActiveChoice=EMT_AVG
  Mux : Mux  Inputs=2
  Ref : Outport
  m : Outport  Port=2
  wires:
  Control loops/2(iqd+-ref) -> Modulation/3(iqd+-*)
  Control loops/1(vqd+-ref) -> Modulation/2(vqd+-*)
  [PQabc] -> Mux/2
  Measurements/5(PQabc) -> [PQabc]
  Modulation/1(Ref) -> Ref/1
  Measurements/4(theta) -> [theta]
  Vabc/1 -> Measurements/1(Vabc)
  Measurements/1(vqd+-) -> Control loops/3(vqd+-), [vqdpn]
  Measurements/2(iqd+-) -> Control loops/4(iqd+-)
  Measurements/3(freq) -> Control loops/5(freq)
  [theta] -> Modulation/4(theta)
  [vqdpn] -> Modulation/1(vqd+-)
  Iabc/1 -> Measurements/2(Iabc)
  Mux/1 -> m/1
  Control loops/3(m) -> Mux/1
  Pset/1 -> Control loops/1(Pset)
  Qset/1 -> Control loops/2(Qset)
  Block/1 -> Control loops/6(Block)

== system EMT_G1/G3/VSC/VSC Model ==
  Ref : Inport
  EMT AVG : Subsystem  VariantControl=EMT_AVG
      settings: PortSchema="{\"entries\":[{\"content\":{\"sides\":[{\"content\":{\"connectorIds\":[\"LConn1\",\"LConn2\",\"LConn3\"]},\"type\":\"ConnectorPlacement.EquallySpacedRectSide\",\"uuid\":\"96043b84-a665-4cb2-a938-d6633d7ee474\"},{\"content\":{\"connectorIds\":[\"In1\"],\"side\":\"RIGHT\"},\"type\":\"ConnectorPlacement.EquallySpacedRectSide\",\"uuid\":\"064d463f-c23a-42ac-89ce-8dea3d446214\"},{\"content\":{\"connectorIds\":[],\"side\":\"TOP\"},\"type\":\"ConnectorPlacement.EquallySpacedRectSide\",\"uuid\":\"95ef669c-c6ed-44c3-8b69-447906728b6d\"}]},\"type\":\"ConnectorPlacement.EquallySpacedConnector\",\"uuid\":\"ea66db09-64d7-4d7e-ba7b-d769c56e2dbd\"}],\"packageUris\":[\"http://schema.mathworks.com/mf0/Connector/19700101\"],\"version\":\"1.0\"}"
  EMT SW : Subsystem  VariantControl=EMT_SW
      settings: PortSchema="{\"entries\":[{\"content\":{\"sides\":[{\"content\":{\"connectorIds\":[\"LConn1\",\"LConn2\",\"LConn3\"]},\"type\":\"ConnectorPlacement.EquallySpacedRectSide\",\"uuid\":\"96043b84-a665-4cb2-a938-d6633d7ee474\"},{\"content\":{\"connectorIds\":[\"In1\"],\"side\":\"RIGHT\"},\"type\":\"ConnectorPlacement.EquallySpacedRectSide\",\"uuid\":\"064d463f-c23a-42ac-89ce-8dea3d446214\"},{\"content\":{\"connectorIds\":[],\"side\":\"TOP\"},\"type\":\"ConnectorPlacement.EquallySpacedRectSide\",\"uuid\":\"95ef669c-c6ed-44c3-8b69-447906728b6d\"}]},\"type\":\"ConnectorPlacement.EquallySpacedConnector\",\"uuid\":\"ea66db09-64d7-4d7e-ba7b-d769c56e2dbd\"}],\"packageUris\":[\"http://schema.mathworks.com/mf0/Connector/19700101\"],\"version\":\"1.0\"}"
  Phasor : Subsystem  VariantControl=Phasor
      settings: PortSchema="{\"entries\":[{\"content\":{\"sides\":[{\"content\":{\"connectorIds\":[\"LConn1\",\"LConn2\",\"LConn3\"]},\"type\":\"ConnectorPlacement.EquallySpacedRectSide\",\"uuid\":\"96043b84-a665-4cb2-a938-d6633d7ee474\"},{\"content\":{\"connectorIds\":[\"In1\"],\"side\":\"RIGHT\"},\"type\":\"ConnectorPlacement.EquallySpacedRectSide\",\"uuid\":\"064d463f-c23a-42ac-89ce-8dea3d446214\"},{\"content\":{\"connectorIds\":[],\"side\":\"TOP\"},\"type\":\"ConnectorPlacement.EquallySpacedRectSide\",\"uuid\":\"95ef669c-c6ed-44c3-8b69-447906728b6d\"}]},\"type\":\"ConnectorPlacement.EquallySpacedConnector\",\"uuid\":\"ea66db09-64d7-4d7e-ba7b-d769c56e2dbd\"}],\"packageUris\":[\"http://schema.mathworks.com/mf0/Connector/19700101\"],\"version\":\"1.0\"}"
  A : PMIOPort  Side=Left
  B : PMIOPort  Port=2  Side=Left
  C : PMIOPort  Port=3  Side=Left

== system EMT_G1/G3/VSC/output signals ==
  Vs : Inport
  Is : Inport  Port=2
  control : Inport  Port=3
  Bus Creator : BusCreator  Inputs=15
  Demux : Demux  Outputs=13
  m : Outport
  wires:
  Bus Creator/1 -> m/1
  control/1 -> Demux/1
  Vs/1 -> Bus Creator/1  "Vabc"
  Is/1 -> Bus Creator/2  "Iabc"
  Demux/1 -> Bus Creator/3  "vqp"
  Demux/2 -> Bus Creator/4  "vdp"
  Demux/3 -> Bus Creator/5  "vqn"
  Demux/4 -> Bus Creator/6  "vdn"
  Demux/5 -> Bus Creator/7  "iqp"
  Demux/6 -> Bus Creator/8  "idp"
  Demux/7 -> Bus Creator/9  "iqn"
  Demux/8 -> Bus Creator/10  "idn"
  Demux/9 -> Bus Creator/11  "f"
  Demux/10 -> Bus Creator/12  "Pdq"
  Demux/11 -> Bus Creator/13  "Qdq"
  Demux/12 -> Bus Creator/14  "Pabc"
  Demux/13 -> Bus Creator/15  "Qabc"

== system EMT_G1/G4s/Exciter System/PSS ==
  note: Power System Stabilizer (PSS2A)
  dw : Inport
  Pgen : Inport  Port=2
  Gain : Gain  Gain=Ks1
  Gain1 : Gain  Gain=Ks3
  Saturation : Saturate  UpperLimit=Vstmax  LowerLimit=Vstmin
  Sum1 : Sum  Inputs=|++
  Sum2 : Sum  Inputs=|+-
  Transfer Fcn1 : TransferFcn  Numerator=[Tw1 0]  Denominator=[Tw1 1]
  Transfer Fcn2 : TransferFcn  Numerator=[Tw3 0]  Denominator=[Tw3 1]
  Transfer Fcn3 : TransferFcn  Numerator=[Tw2 0]  Denominator=[Tw2 1]
  Transfer Fcn4 : TransferFcn  Denominator=[T6 1]
  Transfer Fcn5 : TransferFcn  Numerator=[T8 1].^N  Denominator=[T9 1].^(M*N)
  Transfer Fcn6 : TransferFcn  Numerator=[T1 1]  Denominator=[T2 1]
  Transfer Fcn7 : TransferFcn  Numerator=[T3 1]  Denominator=[T4 1]
  Transfer Fcn8 : TransferFcn  Numerator=[Tw4 0]  Denominator=[Tw4 1]
  Transfer Fcn9 : TransferFcn  Numerator=[Ks2]  Denominator=[T7 1]
  Vothsg : Outport
  wires:
  Transfer Fcn9/1 -> Sum2/2, Gain1/1
  Gain1/1 -> Sum1/2
  Transfer Fcn8/1 -> Transfer Fcn9/1
  Transfer Fcn2/1 -> Transfer Fcn8/1
  Pgen/1 -> Transfer Fcn2/1
  Saturation/1 -> Vothsg/1
  Transfer Fcn7/1 -> Saturation/1
  Transfer Fcn6/1 -> Transfer Fcn7/1
  Gain/1 -> Transfer Fcn6/1
  Sum2/1 -> Gain/1
  Transfer Fcn5/1 -> Sum2/1
  Sum1/1 -> Transfer Fcn5/1
  Transfer Fcn4/1 -> Sum1/1
  Transfer Fcn3/1 -> Transfer Fcn4/1
  Transfer Fcn1/1 -> Transfer Fcn3/1
  dw/1 -> Transfer Fcn1/1

== system EMT_G1/G4s/Exciter System/SEXS ==
  note: The controller parameters provided by ENTSO-E
      | define different names for the parameters:
      |
      | ENTSO-E = IEEE Std 421.5-2005
      | Ta = Tc
      | Tb = Tb
      | K = Ka
      | Te = Ta
      | Emax = Vrmax
      | Emin = Vrmin
  note: The exciter model provided by ENTSO-E most similar to the IEEE is the Type AC4A excitation system model
  Vref : Inport
  Vc : Inport  Port=2
  Vs : Inport  Port=3
  1st ord transfer fcn windup limiter : Subsystem  mask{Gain=K, tau=Te, Vmax=Emax, Vmin=Emin, y0=Vf0}
      mask prompts: tau "Time constant"; y0 "Initial output"
  Constant : Constant  Value=Vf0/K
  Saturation : Saturate  Commented=through  UpperLimit=0.1  LowerLimit=-0.1
  Sum : Sum  Inputs=+-+
  Sum1 : Sum  Inputs=|++
  Transfer Fcn (with initial outputs)1 : simulink_extras/Additional Linear/Transfer Fcn (with initial outputs)  N=[Ta 1]  D=[Tb 1]  Y0=Vf0/K  U0=Vf0/K
  Efd : Outport
  wires:
  1st ord transfer fcn windup limiter/1(Out1) -> Efd/1
  Vs/1 -> Sum/3
  Vref/1 -> Sum/1
  Vc/1 -> Sum/2
  Transfer Fcn (with initial outputs)1/1 -> 1st ord transfer fcn windup limiter/1(In1)
  Saturation/1 -> Transfer Fcn (with initial outputs)1/1
  Sum/1 -> Sum1/1
  Sum1/1 -> Saturation/1
  Constant/1 -> Sum1/2

== system EMT_G1/G4s/Exciter System/TR and LC_test ==
  note: Rc and Xc should be negative values in case of voltage regulated after an impedance
  note: Fig 4.1 of IEEE Std 421.5-2005
  note: Vt and It should be phasors (complex quantities)
  note: compensated
      | impedance
  note: Terminal voltage transducer and optional load compensation
  Vt : Inport
  It : Inport  Port=2
  Abs : Abs  SaturateOnIntegerOverflow=off
  Abs1 : Abs  SaturateOnIntegerOverflow=off
  Rc+jXc : Gain  Gain=abs(Rc+1i*Xc)
  Saturation : Saturate  UpperLimit=1.2  LowerLimit=0.8
  Sum : Sum  Inputs=|+-
  Transfer Fcn (with initial outputs) : simulink_extras/Additional Linear/Transfer Fcn (with initial outputs)  N=[1]  D=[Tr 1]  Y0=1  U0=1
  Vc : Outport
  wires:
  Abs1/1 -> Rc+jXc/1
  Abs/1 -> Sum/1
  It/1 -> Abs1/1
  Sum/1 -> Transfer Fcn (with initial outputs)/1
  Rc+jXc/1 -> Sum/2
  Transfer Fcn (with initial outputs)/1 -> Saturation/1
  Vt/1 -> Abs/1
  Saturation/1 -> Vc/1

== system EMT_G1/G5/VSC/VI measurement ==
  Current Measurement : spsCurrentMeasurementLib/Current Measurement  PhasorSimulation=off  OutputType=Complex  PSBequivalent=0
  Current Measurement1 : spsCurrentMeasurementLib/Current Measurement  PhasorSimulation=off  OutputType=Complex  PSBequivalent=0
  Current Measurement2 : spsCurrentMeasurementLib/Current Measurement  PhasorSimulation=off  OutputType=Complex  PSBequivalent=0
  Ground : spsGroundLib/Ground  LConnTagsString=a
  Ground1 : spsGroundLib/Ground  LConnTagsString=a
  Ground2 : spsGroundLib/Ground  LConnTagsString=a
  Mux : Mux  Inputs=3
  Mux1 : Mux  Inputs=3
  Voltage Measurement : spsVoltageMeasurementLib/Voltage Measurement  PhasorSimulation=off  OutputType=Complex  PSBequivalent=0
  Voltage Measurement1 : spsVoltageMeasurementLib/Voltage Measurement  PhasorSimulation=off  OutputType=Complex  PSBequivalent=0
  Voltage Measurement2 : spsVoltageMeasurementLib/Voltage Measurement  PhasorSimulation=off  OutputType=Complex  PSBequivalent=0
  A : PMIOPort  Side=Left
  B : PMIOPort  Port=2  Side=Left
  C : PMIOPort  Port=3  Side=Left
  a : PMIOPort  Port=4  Side=Right
  b : PMIOPort  Port=5  Side=Right
  c : PMIOPort  Port=6  Side=Right
  Vs : Outport
  Is : Outport  Port=2
  wires:
  Mux1/1 -> Is/1
  Mux/1 -> Vs/1
  Voltage Measurement1/1 -> Mux/2
  Voltage Measurement2/1 -> Mux/3
  Current Measurement2/1 -> Mux1/3
  Voltage Measurement/1 -> Mux/1
  Current Measurement/1 -> Mux1/1
  Current Measurement1/1 -> Mux1/2
  connections:
  Voltage Measurement/LConn1 -- Current Measurement/LConn1 -- A/RConn1
  Current Measurement2/LConn1 -- C/RConn1 -- Voltage Measurement2/LConn1
  Current Measurement1/LConn1 -- Voltage Measurement1/LConn1 -- B/RConn1
  Current Measurement1/RConn1 -- b/RConn1
  Current Measurement/RConn1 -- a/RConn1
  Ground/LConn1 -- Voltage Measurement/LConn2
  Current Measurement2/RConn1 -- c/RConn1
  Ground1/LConn1 -- Voltage Measurement1/LConn2
  Ground2/LConn1 -- Voltage Measurement2/LConn2

== system EMT_G1/G5/VSC/VSC Control ==
  Block : Inport
  Vabc : Inport  Port=2
  Iabc : Inport  Port=3
  Pset : Inport  Port=4
  Qset : Inport  Port=5
  Control loops : Subsystem  Variant=on  VariantControlMode=label  LabelModeActiveChoice=EMT_and_QEMT
  Measurements : Subsystem  Variant=on  VariantControlMode=label  LabelModeActiveChoice=EMT
  Modulation : Subsystem  Variant=on  VariantControlMode=label  LabelModeActiveChoice=EMT_AVG
  Mux : Mux  Inputs=2
  Ref : Outport
  m : Outport  Port=2
  wires:
  Control loops/2(iqd+-ref) -> Modulation/3(iqd+-*)
  Control loops/1(vqd+-ref) -> Modulation/2(vqd+-*)
  [PQabc] -> Mux/2
  Measurements/5(PQabc) -> [PQabc]
  Modulation/1(Ref) -> Ref/1
  Measurements/4(theta) -> [theta]
  Vabc/1 -> Measurements/1(Vabc)
  Measurements/1(vqd+-) -> Control loops/3(vqd+-), [vqdpn]
  Measurements/2(iqd+-) -> Control loops/4(iqd+-)
  Measurements/3(freq) -> Control loops/5(freq)
  [theta] -> Modulation/4(theta)
  [vqdpn] -> Modulation/1(vqd+-)
  Iabc/1 -> Measurements/2(Iabc)
  Mux/1 -> m/1
  Control loops/3(m) -> Mux/1
  Pset/1 -> Control loops/1(Pset)
  Qset/1 -> Control loops/2(Qset)
  Block/1 -> Control loops/6(Block)

== system EMT_G1/G5/VSC/VSC Model ==
  Ref : Inport
  EMT AVG : Subsystem  VariantControl=EMT_AVG
      settings: PortSchema="{\"entries\":[{\"content\":{\"sides\":[{\"content\":{\"connectorIds\":[\"LConn1\",\"LConn2\",\"LConn3\"]},\"type\":\"ConnectorPlacement.EquallySpacedRectSide\",\"uuid\":\"96043b84-a665-4cb2-a938-d6633d7ee474\"},{\"content\":{\"connectorIds\":[\"In1\"],\"side\":\"RIGHT\"},\"type\":\"ConnectorPlacement.EquallySpacedRectSide\",\"uuid\":\"064d463f-c23a-42ac-89ce-8dea3d446214\"},{\"content\":{\"connectorIds\":[],\"side\":\"TOP\"},\"type\":\"ConnectorPlacement.EquallySpacedRectSide\",\"uuid\":\"95ef669c-c6ed-44c3-8b69-447906728b6d\"}]},\"type\":\"ConnectorPlacement.EquallySpacedConnector\",\"uuid\":\"ea66db09-64d7-4d7e-ba7b-d769c56e2dbd\"}],\"packageUris\":[\"http://schema.mathworks.com/mf0/Connector/19700101\"],\"version\":\"1.0\"}"
  EMT SW : Subsystem  VariantControl=EMT_SW
      settings: PortSchema="{\"entries\":[{\"content\":{\"sides\":[{\"content\":{\"connectorIds\":[\"LConn1\",\"LConn2\",\"LConn3\"]},\"type\":\"ConnectorPlacement.EquallySpacedRectSide\",\"uuid\":\"96043b84-a665-4cb2-a938-d6633d7ee474\"},{\"content\":{\"connectorIds\":[\"In1\"],\"side\":\"RIGHT\"},\"type\":\"ConnectorPlacement.EquallySpacedRectSide\",\"uuid\":\"064d463f-c23a-42ac-89ce-8dea3d446214\"},{\"content\":{\"connectorIds\":[],\"side\":\"TOP\"},\"type\":\"ConnectorPlacement.EquallySpacedRectSide\",\"uuid\":\"95ef669c-c6ed-44c3-8b69-447906728b6d\"}]},\"type\":\"ConnectorPlacement.EquallySpacedConnector\",\"uuid\":\"ea66db09-64d7-4d7e-ba7b-d769c56e2dbd\"}],\"packageUris\":[\"http://schema.mathworks.com/mf0/Connector/19700101\"],\"version\":\"1.0\"}"
  Phasor : Subsystem  VariantControl=Phasor
      settings: PortSchema="{\"entries\":[{\"content\":{\"sides\":[{\"content\":{\"connectorIds\":[\"LConn1\",\"LConn2\",\"LConn3\"]},\"type\":\"ConnectorPlacement.EquallySpacedRectSide\",\"uuid\":\"96043b84-a665-4cb2-a938-d6633d7ee474\"},{\"content\":{\"connectorIds\":[\"In1\"],\"side\":\"RIGHT\"},\"type\":\"ConnectorPlacement.EquallySpacedRectSide\",\"uuid\":\"064d463f-c23a-42ac-89ce-8dea3d446214\"},{\"content\":{\"connectorIds\":[],\"side\":\"TOP\"},\"type\":\"ConnectorPlacement.EquallySpacedRectSide\",\"uuid\":\"95ef669c-c6ed-44c3-8b69-447906728b6d\"}]},\"type\":\"ConnectorPlacement.EquallySpacedConnector\",\"uuid\":\"ea66db09-64d7-4d7e-ba7b-d769c56e2dbd\"}],\"packageUris\":[\"http://schema.mathworks.com/mf0/Connector/19700101\"],\"version\":\"1.0\"}"
  A : PMIOPort  Side=Left
  B : PMIOPort  Port=2  Side=Left
  C : PMIOPort  Port=3  Side=Left

== system EMT_G1/G5/VSC/output signals ==
  Vs : Inport
  Is : Inport  Port=2
  control : Inport  Port=3
  Bus Creator : BusCreator  Inputs=15
  Demux : Demux  Outputs=13
  m : Outport
  wires:
  Bus Creator/1 -> m/1
  control/1 -> Demux/1
  Vs/1 -> Bus Creator/1  "Vabc"
  Is/1 -> Bus Creator/2  "Iabc"
  Demux/1 -> Bus Creator/3  "vqp"
  Demux/2 -> Bus Creator/4  "vdp"
  Demux/3 -> Bus Creator/5  "vqn"
  Demux/4 -> Bus Creator/6  "vdn"
  Demux/5 -> Bus Creator/7  "iqp"
  Demux/6 -> Bus Creator/8  "idp"
  Demux/7 -> Bus Creator/9  "iqn"
  Demux/8 -> Bus Creator/10  "idn"
  Demux/9 -> Bus Creator/11  "f"
  Demux/10 -> Bus Creator/12  "Pdq"
  Demux/11 -> Bus Creator/13  "Qdq"
  Demux/12 -> Bus Creator/14  "Pabc"
  Demux/13 -> Bus Creator/15  "Qabc"
